simulink model "RemoteHealthMonitoringSystem"  (R2018a)
settings: Solver=VariableStepAuto  StartTime=0.0  StopTime=inf  RelTol=1e-3
undefined symbols (not defined in the file): ecg_interval, hr_interval, spo2_interval, temp_interval
libraries: arduinolib x2, simulink_extras x1, arduinothingspeaklib x1, instrumentlib x1
settings Model: EnablePacing=on  Creator=Priyadarshi  LastModifiedBy=Priyadarshi

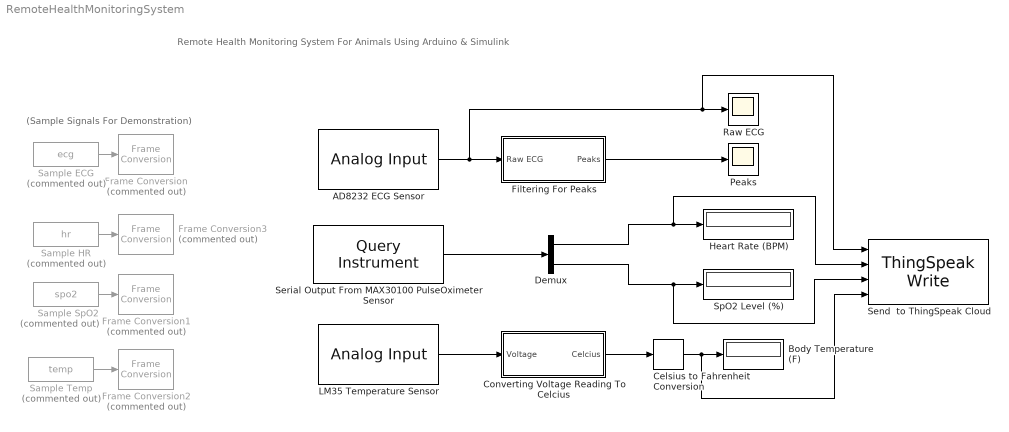
== system RemoteHealthMonitoringSystem ==
  note: (Sample Signals For Demonstration)
  note: Remote Health Monitoring System For Animals Using Arduino & Simulink
  "AD8232 ECG Sensor " : arduinolib/Analog Input  pinNumber=0  ReadResultsOnly=off  ConversionTriggerSource=Software  ExternalTriggerType=uint32(0)  OutputDataType=uint16  EnableConversionCompleteNotify=off  EnableOuputStatus=off  SampleTime=1  blockPlatform=arduino
  "Body Temperature (F) " : Display
  Celsius to Fahrenheit Conversion : simulink_extras/Transformations/Celsius to Fahrenheit
      settings: SourceProductName=Simulink  SourceProductBaseCode=SL
  "Converting Voltage Reading To Celcius " : Subsystem
  Demux : Demux  Outputs=2
  "Filtering For Peaks " : Subsystem
  Frame Conversion{,1..3} (4 alike) : FrameConversion  Commented=on
  Heart Rate (BPM) : Display
  "LM35 Temperature Sensor " : arduinolib/Analog Input  pinNumber=1  ReadResultsOnly=off  ConversionTriggerSource=Software  ExternalTriggerType=uint32(0)  OutputDataType=uint16  EnableConversionCompleteNotify=off  EnableOuputStatus=off  SampleTime=1  blockPlatform=arduino
  "Peaks " : Scope
  Raw ECG : Scope
  Sample ECG : FromWorkspace  Commented=on  VariableName=ecg  SampleTime=ecg_interval
  Sample HR : FromWorkspace  Commented=on  VariableName=hr  SampleTime=hr_interval
  Sample SpO2 : FromWorkspace  Commented=on  VariableName=spo2  SampleTime=spo2_interval
  Sample Temp : FromWorkspace  Commented=on  VariableName=temp  SampleTime=temp_interval
  Send  to ThingSpeak Cloud : arduinothingspeaklib/ThingSpeak Write  ChannelID_=1031010  WriteAPIKey_=Z8TRMAD6TY0RWGY8  NumberOfFields=4  UpdateInterval_=15  PrintDiagnosticMessages_=off  LocationEnabled=off  LocationSource=Block dialog  blockPlatform=arduino  Interfacetype_=Ethernet  UpdateURL=0  StatusMessage=0  StatusEnabled=on  StatusSource=<empty>
      settings: SourceProductName=Simulink Support Package for Arduino Hardware  SourceProductBaseCode=ARDUINO
  Serial Output From MAX30100 PulseOximeter Sensor : instrumentlib/Query Instrument  sampleTime=inf  isWorkspaceObject=off  timeout=10  inputBufferSize=512  protocol=Serial  serialPort=COM1  baudRate=9600  gpibVendor=Keysight Technologies  boardIndex=0  primaryAddress=1  secondaryAddress=0  visaVendor=Keysight  visaSerialPort=0  chassisIndex=0  logicalAddress=0  tcpRemoteHost='127.0.0.1'  tcpRemotePort=4500  udpRemoteHost='127.0.0.1'  udpRemotePort=9090  visaTCPBoardIndex=0  visaTCPRemoteHost='127.0.0.1'  usbBoardIndex=0  usbManufID=0  usbModelCode=0  usbSerialNumber=0  initAction=None  initCommand='DATA:SOURCE CH1'  initFunction=get  queryCommand='curve?'  responseFormat=ASCII  asciiFormatting='%f, %f'  precision=8-bit integer  byteOrder=Little endian  valuesToRead=1  removeBytes=off  afterOutputAction=Repeat query for new data  enableFrames=on  frameSize=2
      settings: SourceProductName=Instrument Control Toolbox  SourceProductBaseCode=IC
  SpO2 Level (%) : Display
  wires:
  "Filtering For Peaks "/1(Peaks) -> "Peaks "/1
  Celsius to Fahrenheit Conversion/1 -> Send  to ThingSpeak Cloud/4, "Body Temperature (F) "/1
  "Converting Voltage Reading To Celcius "/1(Celcius) -> Celsius to Fahrenheit Conversion/1
  "LM35 Temperature Sensor "/1 -> "Converting Voltage Reading To Celcius "/1(Voltage)
  Sample ECG/1 -> Frame Conversion/1
  Sample SpO2/1 -> Frame Conversion1/1
  Sample Temp/1 -> Frame Conversion2/1
  "AD8232 ECG Sensor "/1 -> Send  to ThingSpeak Cloud/1, Raw ECG/1, "Filtering For Peaks "/1(Raw ECG)
  Serial Output From MAX30100 PulseOximeter Sensor/1 -> Demux/1
  Demux/1 -> Send  to ThingSpeak Cloud/2, Heart Rate (BPM)/1
  Demux/2 -> Send  to ThingSpeak Cloud/3, SpO2 Level (%)/1
  Sample HR/1 -> Frame Conversion3/1

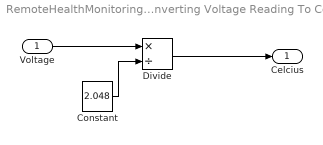
== system RemoteHealthMonitoringSystem/Converting Voltage Reading To Celcius  ==
  Voltage : Inport
  Constant : Constant  Value=2.048
  Divide : Product  Inputs=*/
  Celcius : Outport
  wires:
  Voltage/1 -> Divide/1
  Constant/1 -> Divide/2
  Divide/1 -> Celcius/1

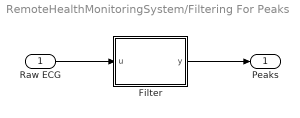
== system RemoteHealthMonitoringSystem/Filtering For Peaks  ==
  Raw ECG : Inport
  Filter : MATLAB Function  TreatAsAtomicUnit=on
  Peaks : Outport
  wires:
  Raw ECG/1 -> Filter/1(u)
  Filter/1(y) -> Peaks/1

== matlab function RemoteHealthMonitoringSystem/Filtering For Peaks /Filter ==
  data: u input; y output
function y = filter(u)
    persistent thres samples
    if isempty(samples)
        samples = cast(0, 'like', u);
        thres = cast(0, 'like', u);
    end
    samples = [samples, u];
    if length(samples)<100
        y = 0;
        return;
    end
    thres = linspace(min(samples), max(samples));
    thres = thres(75);
    y = 0;
    if thres>0
        if u<thres
            y = 0;
        else
            y = u;
        end
    end
end
